simulink model "carsim_cruise_ctrl"  (R2016b)
settings: Solver=ode4  StartTime=0.0  StopTime=30  FixedStep=0.001  RelTol=1e-3
settings Model: Creator=HP  LastModifiedBy=HP

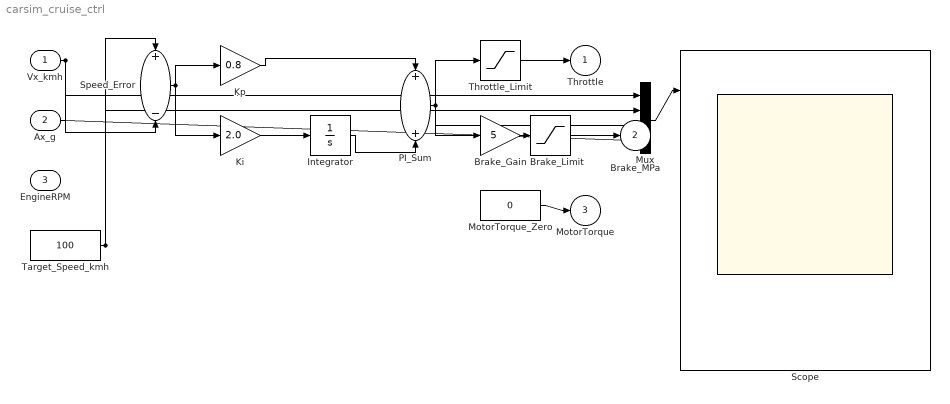
== system carsim_cruise_ctrl ==
  Vx_kmh : Inport
  Ax_g : Inport  Port=2
  EngineRPM : Inport  Port=3
  Brake_Gain : Gain  Gain=5
  Brake_Limit : Saturate  UpperLimit=15  LowerLimit=0
  Integrator : Integrator
  Ki : Gain  Gain=2.0
  Kp : Gain  Gain=0.8
  MotorTorque_Zero : Constant  Value=0
  Mux : Mux
  PI_Sum : Sum
  Scope : Scope  NumInputPorts=4
  Speed_Error : Sum  Inputs=+-
  Target_Speed_kmh : Constant  Value=100
  Throttle_Limit : Saturate  UpperLimit=1  LowerLimit=0
  Throttle : Outport
  Brake_MPa : Outport  Port=2
  MotorTorque : Outport  Port=3
  wires:
  Target_Speed_kmh/1 -> Speed_Error/1, Mux/2
  Vx_kmh/1 -> Speed_Error/2, Mux/1
  Speed_Error/1 -> Kp/1, Ki/1
  Ki/1 -> Integrator/1
  Kp/1 -> PI_Sum/1
  Integrator/1 -> PI_Sum/2
  PI_Sum/1 -> Throttle_Limit/1, Brake_Gain/1, Mux/3
  Throttle_Limit/1 -> Throttle/1
  Brake_Gain/1 -> Brake_Limit/1
  Brake_Limit/1 -> Brake_MPa/1
  MotorTorque_Zero/1 -> MotorTorque/1
  Ax_g/1 -> Mux/4
  Mux/1 -> Scope/1
